simulink model "buckboost_henry"  (R2021b)
settings: Solver=VariableStepAuto  StartTime=0.0  StopTime=.05  RelTol=1e-3
undefined symbols (not defined in the file): C, D, Lminr, Ro, Vin
libraries: spsSeriesRLCBranchLib x3, spsCurrentMeasurementLib x3, spsVoltageMeasurementLib x3, spsMultimeterLib x2, spsDCVoltageSourceLib x1, spsDiodeLib x1, spsMosfetLib x1, simulink x1, spsTriangleGeneratorLib x1, spspowerguiLib x1
settings Model: Creator=Gael Eva  LastModifiedBy=henrysteffens

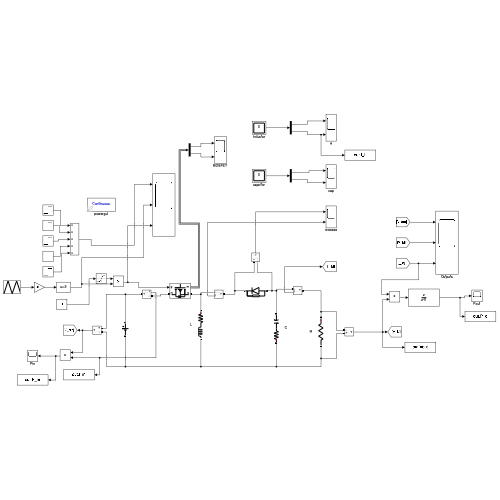
[thumbnail: Simulink's stored preview of the top-level diagram]
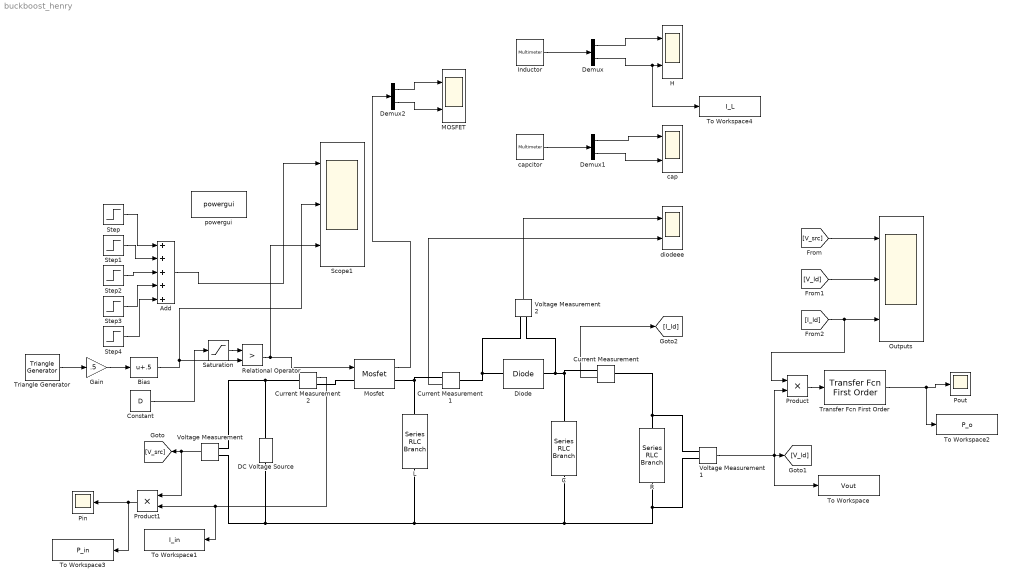
== system buckboost_henry ==
  Add : Sum  Inputs=5
  Bias : Bias  Bias=.5
  C : spsSeriesRLCBranchLib/Series RLC Branch  LConnTagsString=__new0  RConnTagsString=__new0  BranchType=RC  Resistance=4e-3  Inductance=1e-3  SetiL0=off  InitialCurrent=0  Capacitance=C  Setx0=on  InitialVoltage=Vout  Measurements=Branch voltage and current
  Constant : Constant  Value=D
  Current Measurement : spsCurrentMeasurementLib/Current Measurement  PhasorSimulation=off  OutputType=Complex  PSBequivalent=0
  Current Measurement1 : spsCurrentMeasurementLib/Current Measurement  PhasorSimulation=off  OutputType=Complex  PSBequivalent=0
  Current Measurement2 : spsCurrentMeasurementLib/Current Measurement  PhasorSimulation=off  OutputType=Complex  PSBequivalent=0
  DC Voltage Source : spsDCVoltageSourceLib/DC Voltage Source  Amplitude=Vin  Measurements=None
  Demux : Demux  Outputs=2
  Demux1 : Demux  Outputs=2
  Demux2 : Demux  Outputs=2
  Diode : spsDiodeLib/Diode  Ron=0.001  Lon=0  Vf=1.6  IC=0  UseSnubber=0  Rs=500  Cs=250e-9  Measurements=off
  Gain : Gain  Gain=.5
  H : Scope  NumInputPorts=2
  Inductor : spsMultimeterLib/Multimeter  PhasorSimulation=off  OutputType=Complex  sel=[2 4]  L=4  Gain=[1 1]  yselected={'Ub: L','Ib: L'};  PSBOutputType=1  PSBequivalent=0  AxesSetting=[0,0.1,-100,100]  Display=0  SavedBlockNames=-11
  L : spsSeriesRLCBranchLib/Series RLC Branch  LConnTagsString=__new0  RConnTagsString=__new0  BranchType=RL  Resistance=279e-3  Inductance=Lminr  SetiL0=off  InitialCurrent=0  Capacitance=1e-6  Setx0=off  InitialVoltage=0  Measurements=Branch voltage and current
  "MOSFET " : Scope  NumInputPorts=2
  Mosfet : spsMosfetLib/Mosfet  Ron=.75  Lon=0  Rd=0.01  Vfd=0  IC=0  Rs=1e5  Cs=inf  Measurements=on
  Outputs : Scope  NumInputPorts=3
  Pin : Scope
  Pout : Scope
  Product : Product
  Product1 : Product
  R : spsSeriesRLCBranchLib/Series RLC Branch  LConnTagsString=__new0  RConnTagsString=__new0  BranchType=R  Resistance=Ro  Inductance=1e-3  SetiL0=off  InitialCurrent=0  Capacitance=1e-6  Setx0=off  InitialVoltage=0  Measurements=None
  Relational Operator : RelationalOperator  Operator=>  OutDataTypeStr=boolean  RndMeth=Simplest
  Saturation : Saturate  UpperLimit=.9  LowerLimit=0
  Scope1 : Scope  NumInputPorts=3
  Step : Step  After=.05  SampleTime=0
  Step1 : Step  Time=1.25  After=.25  SampleTime=0
  Step2 : Step  Time=1.5  After=.2  SampleTime=0
  Step3 : Step  Time=1.75  After=.25  SampleTime=0
  Step4 : Step  Time=2  After=(.84-.75)  SampleTime=0
  To Workspace : ToWorkspace  VariableName=Vout  SaveFormat=Timeseries  SampleTime=-1
  To Workspace1 : ToWorkspace  VariableName=I_in  SaveFormat=Timeseries  SampleTime=-1
  To Workspace2 : ToWorkspace  VariableName=P_o  SaveFormat=Timeseries  SampleTime=-1
  To Workspace3 : ToWorkspace  VariableName=P_in  SaveFormat=Timeseries  SampleTime=-1
  To Workspace4 : ToWorkspace  VariableName=I_L  SaveFormat=Timeseries  SampleTime=-1
  Transfer Fcn First Order : simulink/Discrete/Transfer Fcn First Order  PoleZ=0  ICPrevOutput=[1, 2*pi*1e3]  DoSatur=off
  Triangle Generator : spsTriangleGeneratorLib/Triangle Generator  Freq=10e3  Phase=0  Ts=0
  Voltage Measurement : spsVoltageMeasurementLib/Voltage Measurement  PhasorSimulation=off  OutputType=Complex  PSBequivalent=0
  Voltage Measurement1 : spsVoltageMeasurementLib/Voltage Measurement  PhasorSimulation=off  OutputType=Complex  PSBequivalent=0
  Voltage Measurement2 : spsVoltageMeasurementLib/Voltage Measurement  PhasorSimulation=off  OutputType=Complex  PSBequivalent=0
  cap : Scope  NumInputPorts=2
  capcitor : spsMultimeterLib/Multimeter  PhasorSimulation=off  OutputType=Complex  sel=[1 3]  L=4  Gain=[1 1]  yselected={'Ub: C','Ib: C'};  PSBOutputType=1  PSBequivalent=0  AxesSetting=[0,0.1,-100,100]  Display=0  SavedBlockNames=-11
  diodeee : Scope  NumInputPorts=2
  powergui : spspowerguiLib/powergui  Priority=1  SimulationMode=Continuous  SampleTime=50e-6  frequency=60  Iterations=50  frequencyindice=0  Pbase=100e6  ErrMax=1e-4  UnitsV=kV  UnitsW=MW  buscounter=0  FunctionMessages=off  echomessages=off  EnableUseOfTLC=off  CurrentSourceSwitches=off  DisableSnubberDevices=off  DisableRonSwitches=off  DisableVfSwitches=off  DisplayEquations=off  AutomaticDiscreteSolvers=off  SolverType=Tustin/Backward Euler (TBE)  Interpol=off  ExternalGateDelay=off  methode=off  Ts=100  x0status=blocks  SPID=on  SwTol=0  HookPort=off  NonlinearTolerance=1e-4  nMaxIteration=100  ContinueOnMaxIteration=off  RestoreLinks=warning  ResistiveCurrentMeasurement=off  Frange=[0:2:500]  Ylog=off  Xlog=on  ShowGrid=off  save=off  variable=ZData  structure=0  ZoomFFT=off  StartTime=0.0  cycles=1  DisplayStyle=1  fundamental=60  FreqAxis=off  MaxFrequency=1000  frequencyindicesteady=1  RmsSteady=1  display=off
  wires:
  Current Measurement/1 -> [I_ld]
  [V_ld] -> Outputs/2
  [V_src] -> Outputs/1
  [I_ld] -> Product/1, Outputs/3
  Gain/1 -> Bias/1
  Step2/1 -> Add/3
  Step1/1 -> Add/2
  Step3/1 -> Add/4
  Step/1 -> Add/1
  Step4/1 -> Add/5
  Add/1 -> Scope1/1
  Relational Operator/1 -> Scope1/3, Mosfet/1
  Bias/1 -> Scope1/2, Relational Operator/2
  Triangle Generator/1 -> Gain/1
  Saturation/1 -> Relational Operator/1
  Voltage Measurement/1 -> Product1/1, [V_src]
  Demux/1 -> H/1
  Inductor/1 -> Demux/1
  capcitor/1 -> Demux1/1
  Demux1/1 -> cap/1
  Demux/2 -> To Workspace4/1, H/2
  Demux1/2 -> cap/2
  Voltage Measurement1/1 -> Product/2, [V_ld], To Workspace/1
  Voltage Measurement2/1 -> diodeee/1
  Constant/1 -> Saturation/1
  Product/1 -> Transfer Fcn First Order/1
  Current Measurement1/1 -> diodeee/2
  Product1/1 -> To Workspace3/1, Pin/1
  Mosfet/1 -> Demux2/1
  Demux2/1 -> "MOSFET "/1
  Demux2/2 -> "MOSFET "/2
  Transfer Fcn First Order/1 -> To Workspace2/1, Pout/1
  Current Measurement2/1 -> To Workspace1/1, Product1/2
  connections:
  DC Voltage Source/RConn1 -- Voltage Measurement/LConn1 -- Current Measurement2/LConn1
  Mosfet/RConn1 -- Current Measurement1/RConn1 -- L/LConn1
  C/RConn1 -- Current Measurement/RConn1 -- Voltage Measurement2/LConn2 -- Diode/LConn1
  R/RConn1 -- Voltage Measurement1/LConn1 -- C/LConn1 -- L/RConn1 -- Voltage Measurement/LConn2 -- DC Voltage Source/LConn1
  Voltage Measurement1/LConn2 -- Current Measurement/LConn1 -- R/LConn1
  Diode/RConn1 -- Current Measurement1/LConn1 -- Voltage Measurement2/LConn1
  Current Measurement2/RConn1 -- Mosfet/LConn1
